simulink model "BirdEyeView_Simulink_intrinsic"  (R2017b)
settings: Solver=FixedStepDiscrete  StartTime=0.0  StopTime=Ts_480p*10  RelTol=1e-3
InitFcn:
  | Ts = 1e-3;
  | Ts_240p = 402*324*Ts;
  | Ts_480p = 525*800*Ts;
undefined symbols (not defined in the file or in its folder): gray, Rec, SDTV
libraries: hdlsllib x7, visionhdlio x2, visionhdlgeotforms x1, visionhdlconversions x1, visiongeotforms x1, dspvision x1
settings Model: DataTypeOverride=Off  ModifiedByFormat=4mbilal@gmail.com  Creator=The MathWorks, Inc.  LastModifiedBy=4mbilal@gmail.com
settings DataIOCC: LimitDataPoints=on  SaveFormat=Array  SaveOutput=off  SaveTime=off
settings OptimizationCC: BlockReduction=off  ConditionallyExecuteInputs=off  DefaultParameterBehavior=Inlined  LifeSpan=inf
settings DebuggingCC: AlgebraicLoopMsg=error  SolverPrmCheckMsg=warning  SingleTaskRateTransMsg=error  ParameterPrecisionLossMsg=none  AllowSymbolicDim=off  SFUnexpectedBacktrackingDiag=warning  SFNoUnconditionalDefaultTransitionDiag=warning  SFExecutionAtInitializationDiag=none  IntegerSaturationMsg=none
settings HardwareCC: ProdBitPerPointer=32  ProdBitPerSizeT=32  ProdBitPerPtrDiffT=32  ProdLargestAtomicFloat=None  ProdIntDivRoundTo=Undefined  ProdEndianess=Unspecified  ProdWordSize=32  ProdHWDeviceType=ASIC/FPGA->ASIC/FPGA  ProdEqTarget=off
settings ModelReferenceCC: PropagateSignalLabelsOutOfModel=off
settings CodeAppCC: StateflowObjectComments=on
settings GRTTargetCC: TargetLangStandard=C89/C90 (ANSI)  GeneratePreprocessorConditionals=Disable all
settings ConfigComp: CovMetricSettings=dw  CovHtmlReporting=on  CovSaveCumulativeToWorkspaceVar=on  CovSaveSingleToWorkspaceVar=on  CovShowResultsExplorer=off  CovExternalEMLEnable=off  CovSFcnEnable=off

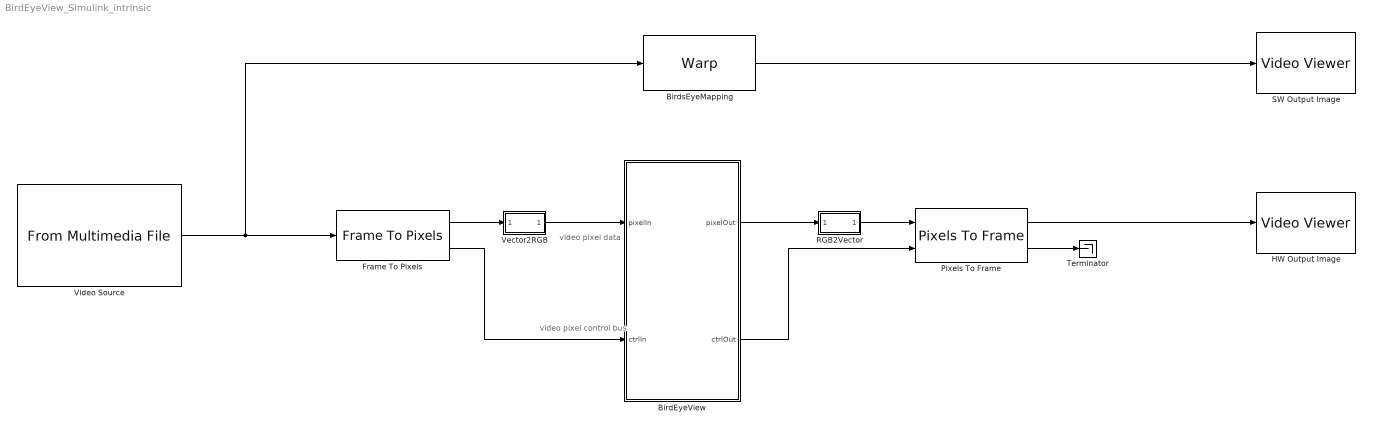
== system BirdEyeView_Simulink_intrinsic ==
  note: video pixel data
  note: video pixel control bus
  BirdEyeView : Subsystem  TreatAsAtomicUnit=on
  BirdsEyeMapping : visiongeotforms/Warp  TransformMatrixSource=Custom  TransformMatrix=[0.000100990123328 0 0;0.000412396945637 0.001302203393162 1.293171994e-06;-0.103019798961327 -0.255811259450009 -0.000222053779501]  InterpolationMethod=Nearest neighbor  BackgroundFillValue=0  OutputImagePositionSource=Custom  OutputImagePosition=[ 1, 1, 640, 480 ]  ROIInputPort=off  ROIValidityOutputPort=off  SimulateUsing=Code generation
      settings: SourceProductName=Computer Vision System Toolbox  SourceProductBaseCode=VP
  Frame To Pixels : visionhdlio/Frame To Pixels  NumComponents=3  VideoFormat=480p  ActivePixelsPerLine=32  ActiveVideoLines=18  TotalPixelsPerLine=42  TotalVideoLines=28  StartingActiveLine=6  FrontPorch=5  SampleTime=0
      settings: SourceProductName=Vision HDL Toolbox  SourceProductBaseCode=VT
  HW Output Image : VideoViewer  colormapValue=gray(256)  FigPos=[769.8 637.2 730.4 446.4]
  Pixels To Frame : visionhdlio/Pixels To Frame  NumComponents=3  VideoFormat=480p  ActivePixelsPerLine=32  ActiveVideoLines=18  TotalPixelsPerLine=42  TotalVideoLines=28
      settings: SourceProductName=Vision HDL Toolbox  SourceProductBaseCode=VT
  RGB2Vector : Subsystem
  SW Output Image : VideoViewer  colormapValue=gray(256)  FigPos=[62.6 646 730.4 446.4]
  Terminator : Terminator
  Vector2RGB : Subsystem
  Video Source : dspvision/From Multimedia File  inputFilename=E:\RnD\Current_Projects\Musawwir\Frameworks\HW\Musawwir_HW_Zedboard\Custom_IP_Cores\Matlab\LaneDetection\test.jpg  loop=on  numPlays=inf  outputStreams=Video only  videoDataType=uint8  audioDataType=int16  inheritSampleTime=off  userDefinedSampleTime=Ts_480p  noAudioOutput=off  isIntensityVideo=off  fourcc=RGB  colorVideoFormat=One multidimensional signal  outputEOF=off  dataOrg=Column-major  audioFrameSize=1024  computeAudioFrameSize=off  outSamplingMode=Sample based
      settings: SourceProductBaseCode=VP
  wires:
  Pixels To Frame/2 -> Terminator/1
  Vector2RGB/1(RGB) -> BirdEyeView/1(pixelIn)
  BirdEyeView/1(pixelOut) -> RGB2Vector/1(RGB)
  Frame To Pixels/1 -> Vector2RGB/1(RGBVector)
  BirdEyeView/2(ctrlOut) -> Pixels To Frame/2
  Frame To Pixels/2 -> BirdEyeView/2(ctrlIn)
  RGB2Vector/1(RGBVector) -> Pixels To Frame/1
  Video Source/1 -> BirdsEyeMapping/1, Frame To Pixels/1
  Pixels To Frame/1 -> HW Output Image/1
  BirdsEyeMapping/1 -> SW Output Image/1

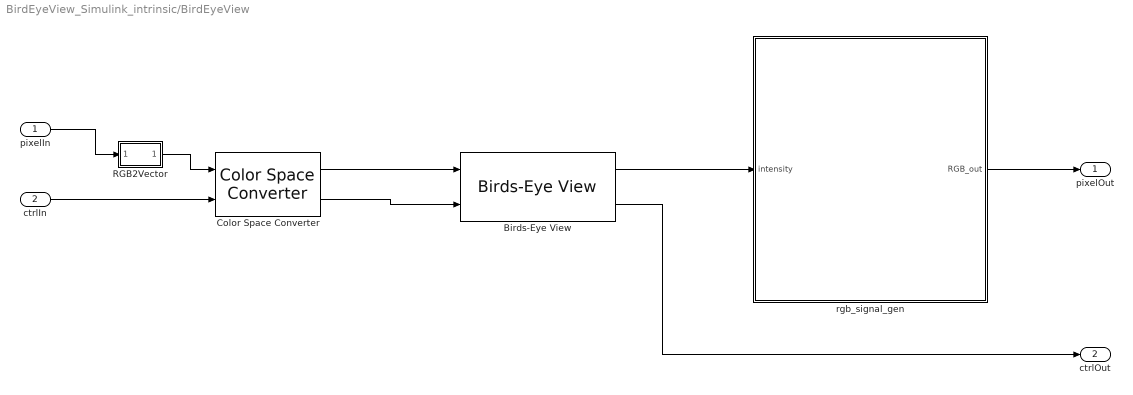
== system BirdEyeView_Simulink_intrinsic/BirdEyeView ==
  pixelIn : Inport
  ctrlIn : Inport  Port=2
  Birds-Eye View : visionhdlgeotforms/Birds-Eye View  HomographyMatrix=[0.000100990123328 0 0;0.000412396945637 0.001302203393162 1.293171994e-06;-0.103019798961327 -0.255811259450009 -0.000222053779501]  MaxBufferSize=40000  MaxSourceLinesBuffered=54  BirdsEyeActivePixels=640  BirdsEyeActiveLines=480  SimulateUsing=Code generation
      settings: SourceProductName=Vision HDL Toolbox  SourceProductBaseCode=VT
  Color Space Converter : visionhdlconversions/Color Space Converter  Conversion=RGB to intensity  ConversionStandard=Rec. 601 (SDTV)  ScanningStandard=1250/50/2:1  SimulateUsing=Code generation
      settings: SourceProductName=Vision HDL Toolbox  SourceProductBaseCode=VT
  RGB2Vector : Subsystem
  rgb_signal_gen : MATLAB Function  TreatAsAtomicUnit=on
  pixelOut : Outport
  ctrlOut : Outport  Port=2
  wires:
  ctrlIn/1 -> Color Space Converter/2
  pixelIn/1 -> RGB2Vector/1(RGB)
  RGB2Vector/1(RGBVector) -> Color Space Converter/1
  rgb_signal_gen/1(RGB_out) -> pixelOut/1
  Color Space Converter/1 -> Birds-Eye View/1
  Birds-Eye View/1 -> rgb_signal_gen/1(intensity)
  Color Space Converter/2 -> Birds-Eye View/2
  Birds-Eye View/2 -> ctrlOut/1

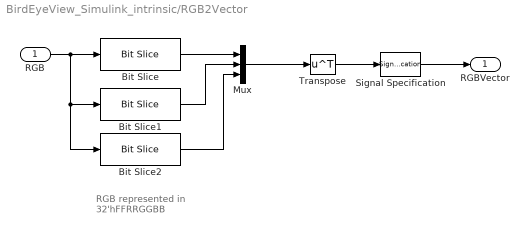
== system BirdEyeView_Simulink_intrinsic/RGB2Vector ==
  note: RGB represented in
      | 32'hFFRRGGBB
  RGB : Inport
  Bit Slice : hdlsllib/Logic and Bit Operations/Bit Slice  lidx=23  ridx=16
  Bit Slice1 : hdlsllib/Logic and Bit Operations/Bit Slice  lidx=15  ridx=8
  Bit Slice2 : hdlsllib/Logic and Bit Operations/Bit Slice  lidx=7  ridx=0
  Mux : Mux  Inputs=3
  Signal Specification : SignalSpecification
  Transpose : Math  Operator=transpose  SaturateOnIntegerOverflow=on
  RGBVector : Outport
  wires:
  Mux/1 -> Transpose/1
  Bit Slice/1 -> Mux/1
  Bit Slice2/1 -> Mux/3
  Bit Slice1/1 -> Mux/2
  RGB/1 -> Bit Slice2/1, Bit Slice1/1, Bit Slice/1
  Transpose/1 -> Signal Specification/1
  Signal Specification/1 -> RGBVector/1

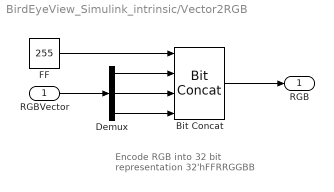
== system BirdEyeView_Simulink_intrinsic/Vector2RGB ==
  note: Encode RGB into 32 bit representation
      | 32'hFFRRGGBB
  RGBVector : Inport
  Bit Concat : hdlsllib/Logic and Bit Operations/Bit Concat  numInputs=4
      settings: SourceProductName=HDL Coder  SourceProductBaseCode=HD
  Demux : Demux  Outputs=3
  FF : Constant  Value=255  OutDataTypeStr=uint8  SampleTime=Ts
  RGB : Outport
  wires:
  Bit Concat/1 -> RGB/1
  RGBVector/1 -> Demux/1
  FF/1 -> Bit Concat/1
  Demux/1 -> Bit Concat/2
  Demux/2 -> Bit Concat/3
  Demux/3 -> Bit Concat/4

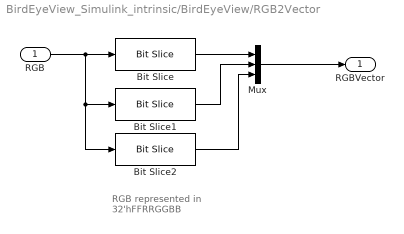
== system BirdEyeView_Simulink_intrinsic/BirdEyeView/RGB2Vector ==
  note: RGB represented in
      | 32'hFFRRGGBB
  RGB : Inport
  Bit Slice : hdlsllib/Logic and Bit Operations/Bit Slice  lidx=23  ridx=16
  Bit Slice1 : hdlsllib/Logic and Bit Operations/Bit Slice  lidx=15  ridx=8
  Bit Slice2 : hdlsllib/Logic and Bit Operations/Bit Slice  lidx=7  ridx=0
  Mux : Mux  Inputs=3
  RGBVector : Outport
  wires:
  Bit Slice/1 -> Mux/1
  Bit Slice2/1 -> Mux/3
  Bit Slice1/1 -> Mux/2
  RGB/1 -> Bit Slice2/1, Bit Slice1/1, Bit Slice/1
  Mux/1 -> RGBVector/1

== matlab function BirdEyeView_Simulink_intrinsic/BirdEyeView/rgb_signal_gen ==
  data: intensity input; RGB_out output
function RGB_out  = rgb_signal_gen(intensity)

in_d = double(intensity);%Double precision format
% in_d = double(bypass);%Double precision format

R = fi(in_d, 0, 8, 0);%convert to fixed-point 8-bit signal
G = fi(in_d, 0, 8, 0);
B = fi(in_d, 0, 8, 0);
A = fi(255, 0, 8, 0);

RGB_out = bitconcat(A,R,G,B);%32-bit output signal
